simulink library "utilities"  (R2024a)
settings: Solver=VariableStepAuto  StartTime=0.0  StopTime=10.0  RelTol=1e-3
settings Model: Creator=imyrsini  LastModifiedBy=imyrsini

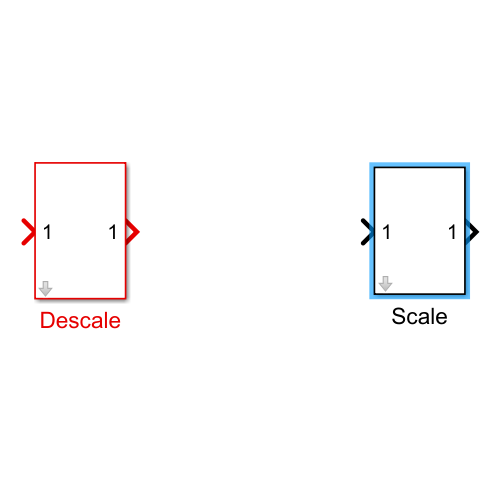
[thumbnail: Simulink's stored preview of the top-level diagram]
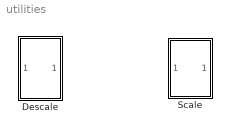
== system utilities ==
  Descale : Subsystem  mask{Std=0, Mean=0}
      mask prompts: Std "Standard deviation"; Mean "Mean value"
  Scale : Subsystem  mask{Std=0, Mean=0}
      mask prompts: Std "Standard deviation"; Mean "Mean value"

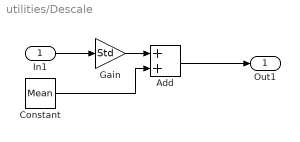
== system utilities/Descale ==
  In1 : Inport
  Add : Sum
  Constant : Constant  Value=Mean
  Gain : Gain  Gain=Std
  Out1 : Outport
  wires:
  Constant/1 -> Add/2
  Gain/1 -> Add/1
  Add/1 -> Out1/1
  In1/1 -> Gain/1

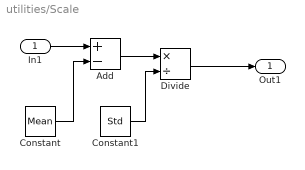
== system utilities/Scale ==
  In1 : Inport
  Add : Sum  Inputs=+-
  Constant : Constant  Value=Mean
  Constant1 : Constant  Value=Std
  Divide : Product  Inputs=*/
  Out1 : Outport
  wires:
  In1/1 -> Add/1
  Constant/1 -> Add/2
  Add/1 -> Divide/1
  Divide/1 -> Out1/1
  Constant1/1 -> Divide/2
